simulink model "Voltage_and_Current_Measurement_MTL__18032026"  (R2024b)
settings: Solver=VariableStepAuto  StartTime=0.0  StopTime=10.0  RelTol=1e-3
libraries: spsThreePhaseVIMeasurementLib x12, spsRMSLib x8, spsThreePhasePISectionLineLib x6, spsThreePhaseSeriesRLCBranchLib x6, spsThreePhaseSourceLib x6, sps_lib x5, spsPower3phInstantaneousLib x4, spsGroundLib x3, spsThreePhaseSeriesRLCLoadLib x2, spsThreePhaseParallelRLCBranchLib x1
settings Model: Creator=cachu  LastModifiedBy=cachu

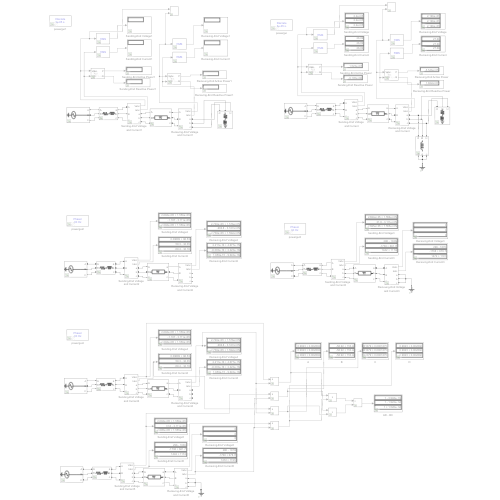
[thumbnail: Simulink's stored preview of the top-level diagram]
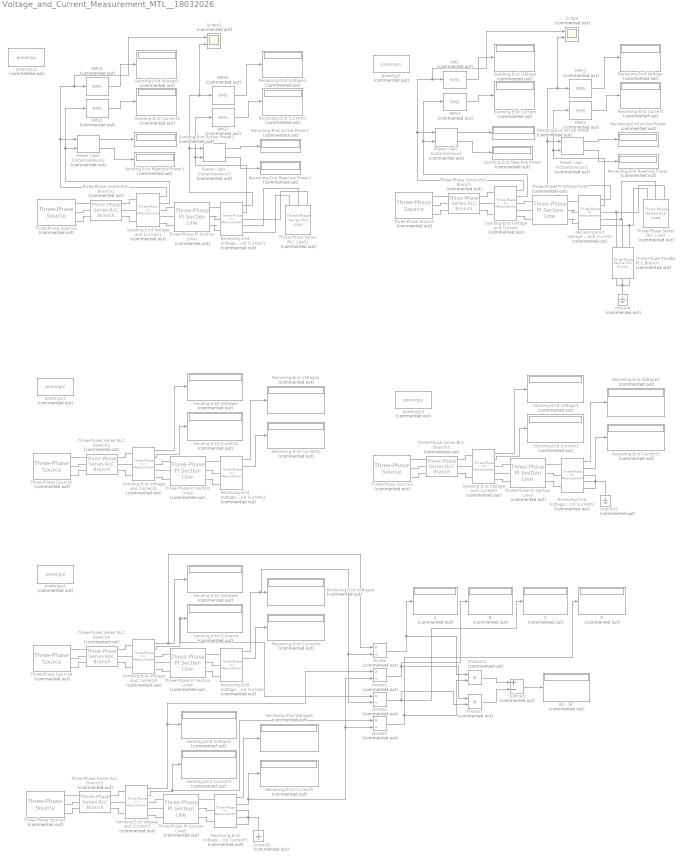
== system Voltage_and_Current_Measurement_MTL__18032026 ==
  A : Display  Commented=on
  AD - BC : Display  Commented=on
  B : Display  Commented=on
  C : Display  Commented=on
  D : Display  Commented=on
  Divide{,1..3} (4 alike) : Product  Commented=on  Inputs=*/
  Ground : spsGroundLib/Ground  Commented=on  LConnTagsString=a
  Ground1 : spsGroundLib/Ground  Commented=on  LConnTagsString=a
  Ground2 : spsGroundLib/Ground  Commented=on  LConnTagsString=a
  Power (3ph, Instantaneous){,1..3} (4 alike) : spsPower3phInstantaneousLib/Power (3ph, Instantaneous)  Commented=on
  Product : Product  Commented=on
  Product1 : Product  Commented=on
  RMS{,1..7} (8 alike) : spsRMSLib/RMS  Commented=on  TrueRMS=on  Freq=50  RMSInit=120  Ts=0
  Recieving-End Active Power : Display  Commented=on
  Recieving-End Active Power1 : Display  Commented=on
  Recieving-End Current{,1..5} (6 alike) : Display  Commented=on
  Recieving-End Reactive Power : Display  Commented=on
  Recieving-End Reactive Power1 : Display  Commented=on
  Recieving-End Voltage{,1..5} (6 alike) : Display  Commented=on
  Recieving-End Voltage and Current{,1,4..5} (4 alike) : spsThreePhaseVIMeasurementLib/Three-Phase V-I Measurement  Commented=on  VoltageMeasurement=phase-to-phase  SetLabelV=off  LabelV=Vabc  Vpu=off  VpuLL=off  CurrentMeasurement=yes  SetLabelI=off  LabelI=Iabc  Ipu=off  Pbase=100e6  Vbase=500e3  OutputType=Complex  PhasorSimulation=off  PSBequivalent=0
  Recieving-End Voltage and Current2 : spsThreePhaseVIMeasurementLib/Three-Phase V-I Measurement  Commented=on  VoltageMeasurement=phase-to-phase  SetLabelV=off  LabelV=Vabc  Vpu=off  VpuLL=off  CurrentMeasurement=yes  SetLabelI=off  LabelI=Iabc  Ipu=off  Pbase=100e6  Vbase=500e3  OutputType=Complex  PhasorSimulation=on  PSBequivalent=0
  Recieving-End Voltage and Current3 : spsThreePhaseVIMeasurementLib/Three-Phase V-I Measurement  Commented=on  VoltageMeasurement=phase-to-phase  SetLabelV=off  LabelV=Vabc  Vpu=off  VpuLL=off  CurrentMeasurement=yes  SetLabelI=off  LabelI=Iabc  Ipu=off  Pbase=100e6  Vbase=500e3  OutputType=Complex  PhasorSimulation=on  PSBequivalent=0
  Scope : Scope  Commented=on  NumInputPorts=2
  Scope1 : Scope  Commented=on  NumInputPorts=2
  Sending-End Active Power : Display  Commented=on
  Sending-End Active Power1 : Display  Commented=on
  Sending-End Current{,1..5} (6 alike) : Display  Commented=on
  Sending-End Reactive Power : Display  Commented=on
  Sending-End Reactive Power1 : Display  Commented=on
  Sending-End Voltage{,1..5} (6 alike) : Display  Commented=on
  Sending-End Voltage and Current{,1,4..5} (4 alike) : spsThreePhaseVIMeasurementLib/Three-Phase V-I Measurement  Commented=on  VoltageMeasurement=phase-to-phase  SetLabelV=off  LabelV=Vabc  Vpu=off  VpuLL=off  CurrentMeasurement=yes  SetLabelI=off  LabelI=Iabc  Ipu=off  Pbase=100e6  Vbase=500e3  OutputType=Complex  PhasorSimulation=off  PSBequivalent=0
  Sending-End Voltage and Current2 : spsThreePhaseVIMeasurementLib/Three-Phase V-I Measurement  Commented=on  VoltageMeasurement=phase-to-phase  SetLabelV=off  LabelV=Vabc  Vpu=off  VpuLL=off  CurrentMeasurement=yes  SetLabelI=off  LabelI=Iabc  Ipu=off  Pbase=100e6  Vbase=500e3  OutputType=Complex  PhasorSimulation=on  PSBequivalent=0
  Sending-End Voltage and Current3 : spsThreePhaseVIMeasurementLib/Three-Phase V-I Measurement  Commented=on  VoltageMeasurement=phase-to-phase  SetLabelV=off  LabelV=Vabc  Vpu=off  VpuLL=off  CurrentMeasurement=yes  SetLabelI=off  LabelI=Iabc  Ipu=off  Pbase=100e6  Vbase=500e3  OutputType=Complex  PhasorSimulation=on  PSBequivalent=0
  Subtract : Sum  Commented=on  Inputs=+-
  Three-Phase PI Section Line{,1..5} (6 alike) : spsThreePhasePISectionLineLib/Three-Phase PI Section Line  Commented=on  LConnTagsString=a|b|c  RConnTagsString=A|B|C  Length=150  Frequency=50  Resistances=[0.1 0.2]  Inductances=[2e-3 4e-3]  Capacitances=[8e-9 16e-9]
  Three-Phase Parallel RLC Branch : spsThreePhaseParallelRLCBranchLib/Three-Phase Parallel RLC Branch  Commented=on  LConnTagsString=A|B|C  RConnTagsString=A|B|C  BranchType=L  Resistance=0  Inductance=20  Capacitance=0  Measurements=None
  Three-Phase Series RLC Branch{,1..5} (6 alike) : spsThreePhaseSeriesRLCBranchLib/Three-Phase Series RLC Branch  Commented=on  LConnTagsString=A|B|C  RConnTagsString=A|B|C  BranchType=RL  Resistance=0.01  Inductance=1e-12  Capacitance=1e-6  Measurements=None
  Three-Phase Series RLC Load : spsThreePhaseSeriesRLCLoadLib/Three-Phase Series RLC Load  Commented=on  LConnTagsString=A|B|C  Configuration=Y (grounded)  NominalVoltage=220e3  Vabc=[1e3 1e3 1e3]  Vabcp=[1e3 1e3 1e3]  NominalFrequency=50  UnbalancedPower=off  ActivePower=5e6  InductivePower=1.6e6  CapacitivePower=0  Pabc=[10e3 9e3 11e3]  QLabc=[100 90 110]  QCabc=[100 90 110]  Pabcp=[10e3 9e3 11e3]  QLabcp=[100 90 110]  QCabcp=[100 90 110]  Measurements=None  LoadType=constant Z
  Three-Phase Series RLC Load1 : spsThreePhaseSeriesRLCLoadLib/Three-Phase Series RLC Load  Commented=on  LConnTagsString=A|B|C  Configuration=Y (grounded)  NominalVoltage=220e3  Vabc=[1e3 1e3 1e3]  Vabcp=[1e3 1e3 1e3]  NominalFrequency=50  UnbalancedPower=off  ActivePower=5e6  InductivePower=1.6e6  CapacitivePower=0  Pabc=[10e3 9e3 11e3]  QLabc=[100 90 110]  QCabc=[100 90 110]  Pabcp=[10e3 9e3 11e3]  QLabcp=[100 90 110]  QCabcp=[100 90 110]  Measurements=None  LoadType=constant Z
  Three-Phase Source{,1..5} (6 alike) : spsThreePhaseSourceLib/Three-Phase Source  Commented=on  InternalConnection=Yg  VoltagePhases=off  Voltage=220e3  PhaseAngle=0  Voltage_phases=[25e3 25e3 25e3]/sqrt(3)  PhaseAngles_phases=[0 -120 +120]  Frequency=50  NonIdealSource=off  SpecifyImpedance=off  Resistance=0.8929  Inductance=16.58e-3  ShortCircuitLevel=100e6  BaseVoltage=25e3  XRratio=7  BusType=swing  Pref=10e3  Qref=0  Prefabc=[10e3, 10e3, 10e3]  Qrefabc=[0, 0, 0]  Qmin=-inf  Qmax=inf
  powergui : sps_lib/powergui  Priority=1  Commented=on  SimulationMode=Discrete  SampleTime=50e-6  frequency=50  Iterations=50  frequencyindice=50  Pbase=100e6  ErrMax=1e-4  UnitsV=kV  UnitsW=MW  buscounter=0  FunctionMessages=off  echomessages=off  EnableUseOfTLC=off  CurrentSourceSwitches=off  DisableSnubberDevices=off  DisableRonSwitches=off  DisableVfSwitches=off  DisplayEquations=off  AutomaticDiscreteSolvers=off  SolverType=Tustin/Backward Euler (TBE)  Interpol=off  ExternalGateDelay=off  methode=off  Ts=100  x0status=blocks  SPID=on  SwTol=0  HookPort=off  NonlinearTolerance=1e-4  nMaxIteration=100  ContinueOnMaxIteration=off  RestoreLinks=warning  ResistiveCurrentMeasurement=off  Frange=[0:2:500]  Ylog=off  Xlog=on  ShowGrid=off  save=off  variable=ZData  structure=0  ZoomFFT=off  StartTime=0.0  cycles=1  DisplayStyle=1  fundamental=60  FreqAxis=off  MaxFrequency=1000  frequencyindicesteady=1  RmsSteady=1  display=off
  powergui1 : sps_lib/powergui  Priority=1  Commented=on  SimulationMode=Discrete  SampleTime=50e-6  frequency=50  Iterations=50  frequencyindice=50  Pbase=100e6  ErrMax=1e-4  UnitsV=kV  UnitsW=MW  buscounter=0  FunctionMessages=off  echomessages=off  EnableUseOfTLC=off  CurrentSourceSwitches=off  DisableSnubberDevices=off  DisableRonSwitches=off  DisableVfSwitches=off  DisplayEquations=off  AutomaticDiscreteSolvers=off  SolverType=Tustin/Backward Euler (TBE)  Interpol=off  ExternalGateDelay=off  methode=off  Ts=100  x0status=blocks  SPID=on  SwTol=0  HookPort=off  NonlinearTolerance=1e-4  nMaxIteration=100  ContinueOnMaxIteration=off  RestoreLinks=warning  ResistiveCurrentMeasurement=off  Frange=[0:2:500]  Ylog=off  Xlog=on  ShowGrid=off  save=off  variable=ZData  structure=0  ZoomFFT=off  StartTime=0.0  cycles=1  DisplayStyle=1  fundamental=60  FreqAxis=off  MaxFrequency=1000  frequencyindicesteady=1  RmsSteady=1  display=off
  powergui2 : sps_lib/powergui  Priority=1  Commented=on  SimulationMode=Phasor  SampleTime=50e-6  frequency=50  Iterations=50  frequencyindice=50  Pbase=100e6  ErrMax=1e-4  UnitsV=kV  UnitsW=MW  buscounter=0  FunctionMessages=off  echomessages=off  EnableUseOfTLC=off  CurrentSourceSwitches=off  DisableSnubberDevices=off  DisableRonSwitches=off  DisableVfSwitches=off  DisplayEquations=off  AutomaticDiscreteSolvers=off  SolverType=Tustin/Backward Euler (TBE)  Interpol=off  ExternalGateDelay=off  methode=off  Ts=100  x0status=blocks  SPID=on  SwTol=0  HookPort=off  NonlinearTolerance=1e-4  nMaxIteration=100  ContinueOnMaxIteration=off  RestoreLinks=warning  ResistiveCurrentMeasurement=off  Frange=[0:2:500]  Ylog=off  Xlog=on  ShowGrid=off  save=off  variable=ZData  structure=0  ZoomFFT=off  StartTime=0.0  cycles=1  DisplayStyle=1  fundamental=60  FreqAxis=off  MaxFrequency=1000  frequencyindicesteady=1  RmsSteady=1  display=off
  powergui3 : sps_lib/powergui  Priority=1  Commented=on  SimulationMode=Phasor  SampleTime=50e-6  frequency=50  Iterations=50  frequencyindice=50  Pbase=100e6  ErrMax=1e-4  UnitsV=kV  UnitsW=MW  buscounter=0  FunctionMessages=off  echomessages=off  EnableUseOfTLC=off  CurrentSourceSwitches=off  DisableSnubberDevices=off  DisableRonSwitches=off  DisableVfSwitches=off  DisplayEquations=off  AutomaticDiscreteSolvers=off  SolverType=Tustin/Backward Euler (TBE)  Interpol=off  ExternalGateDelay=off  methode=off  Ts=100  x0status=blocks  SPID=on  SwTol=0  HookPort=off  NonlinearTolerance=1e-4  nMaxIteration=100  ContinueOnMaxIteration=off  RestoreLinks=warning  ResistiveCurrentMeasurement=off  Frange=[0:2:500]  Ylog=off  Xlog=on  ShowGrid=off  save=off  variable=ZData  structure=0  ZoomFFT=off  StartTime=0.0  cycles=1  DisplayStyle=1  fundamental=60  FreqAxis=off  MaxFrequency=1000  frequencyindicesteady=1  RmsSteady=1  display=off
  powergui4 : sps_lib/powergui  Priority=1  Commented=on  SimulationMode=Phasor  SampleTime=50e-6  frequency=50  Iterations=50  frequencyindice=50  Pbase=100e6  ErrMax=1e-4  UnitsV=kV  UnitsW=MW  buscounter=0  FunctionMessages=off  echomessages=off  EnableUseOfTLC=off  CurrentSourceSwitches=off  DisableSnubberDevices=off  DisableRonSwitches=off  DisableVfSwitches=off  DisplayEquations=off  AutomaticDiscreteSolvers=off  SolverType=Tustin/Backward Euler (TBE)  Interpol=off  ExternalGateDelay=off  methode=off  Ts=100  x0status=blocks  SPID=on  SwTol=0  HookPort=off  NonlinearTolerance=1e-4  nMaxIteration=100  ContinueOnMaxIteration=off  RestoreLinks=warning  ResistiveCurrentMeasurement=off  Frange=[0:2:500]  Ylog=off  Xlog=on  ShowGrid=off  save=off  variable=ZData  structure=0  ZoomFFT=off  StartTime=0.0  cycles=1  DisplayStyle=1  fundamental=60  FreqAxis=off  MaxFrequency=1000  frequencyindicesteady=1  RmsSteady=1  display=off
  wires:
  RMS/1 -> Sending-End Voltage/1
  Sending-End Voltage and Current/1 -> "Power (3ph, Instantaneous)"/1, Scope/1, RMS/1
  Sending-End Voltage and Current/2 -> RMS1/1, "Power (3ph, Instantaneous)"/2
  RMS1/1 -> Sending-End Current/1
  "Power (3ph, Instantaneous)"/2 -> Sending-End Reactive Power/1
  "Power (3ph, Instantaneous)"/1 -> Sending-End Active Power/1
  Recieving-End Voltage and Current/1 -> Scope/2, RMS2/1, "Power (3ph, Instantaneous)1"/1
  Recieving-End Voltage and Current/2 -> RMS3/1, "Power (3ph, Instantaneous)1"/2
  "Power (3ph, Instantaneous)1"/1 -> Recieving-End Active Power/1
  RMS3/1 -> Recieving-End Current/1
  RMS2/1 -> Recieving-End Voltage/1
  "Power (3ph, Instantaneous)1"/2 -> Recieving-End Reactive Power/1
  Sending-End Voltage and Current1/1 -> "Power (3ph, Instantaneous)2"/1, Scope1/1, RMS4/1
  Recieving-End Voltage and Current1/1 -> Scope1/2, RMS6/1, "Power (3ph, Instantaneous)3"/1
  "Power (3ph, Instantaneous)2"/1 -> Sending-End Active Power1/1
  RMS4/1 -> Sending-End Voltage1/1
  "Power (3ph, Instantaneous)2"/2 -> Sending-End Reactive Power1/1
  RMS7/1 -> Recieving-End Current1/1
  RMS6/1 -> Recieving-End Voltage1/1
  Recieving-End Voltage and Current1/2 -> RMS7/1, "Power (3ph, Instantaneous)3"/2
  "Power (3ph, Instantaneous)3"/2 -> Recieving-End Reactive Power1/1
  "Power (3ph, Instantaneous)3"/1 -> Recieving-End Active Power1/1
  Sending-End Voltage and Current1/2 -> RMS5/1, "Power (3ph, Instantaneous)2"/2
  RMS5/1 -> Sending-End Current1/1
  Recieving-End Voltage and Current2/1 -> Recieving-End Voltage2/1
  Recieving-End Voltage and Current2/2 -> Recieving-End Current2/1
  Sending-End Voltage and Current2/1 -> Sending-End Voltage2/1
  Sending-End Voltage and Current2/2 -> Sending-End Current2/1
  Recieving-End Voltage and Current3/1 -> Recieving-End Voltage3/1
  Recieving-End Voltage and Current3/2 -> Recieving-End Current3/1
  Sending-End Voltage and Current3/2 -> Sending-End Current3/1
  Sending-End Voltage and Current3/1 -> Sending-End Voltage3/1
  Sending-End Voltage and Current5/1 -> Divide1/1, Sending-End Voltage5/1
  Sending-End Voltage and Current5/2 -> Divide3/1, Sending-End Current5/1
  Recieving-End Voltage and Current4/1 -> Divide2/2, Divide/2, Recieving-End Voltage4/1
  Recieving-End Voltage and Current4/2 -> Recieving-End Current4/1
  Sending-End Voltage and Current4/2 -> Divide2/1, Sending-End Current4/1
  Sending-End Voltage and Current4/1 -> Divide/1, Sending-End Voltage4/1
  Recieving-End Voltage and Current5/1 -> Recieving-End Voltage5/1
  Recieving-End Voltage and Current5/2 -> Divide1/2, Divide3/2, Recieving-End Current5/1
  Divide/1 -> Product1/1, A/1
  Divide1/1 -> Product/1, B/1
  Divide2/1 -> Product/2, C/1
  Divide3/1 -> Product1/2, D/1
  Subtract/1 -> AD - BC/1
  Product1/1 -> Subtract/1
  Product/1 -> Subtract/2
  connections:
  Sending-End Voltage and Current/RConn1 -- Three-Phase PI Section Line/LConn1
  Sending-End Voltage and Current/RConn2 -- Three-Phase PI Section Line/LConn2
  Sending-End Voltage and Current/RConn3 -- Three-Phase PI Section Line/LConn3
  Recieving-End Voltage and Current/LConn1 -- Three-Phase PI Section Line/RConn1
  Three-Phase PI Section Line/RConn2 -- Recieving-End Voltage and Current/LConn2
  Three-Phase PI Section Line/RConn3 -- Recieving-End Voltage and Current/LConn3
  Three-Phase Series RLC Load/LConn1 -- Recieving-End Voltage and Current/RConn3 -- Three-Phase Parallel RLC Branch/LConn3
  Recieving-End Voltage and Current/RConn2 -- Three-Phase Parallel RLC Branch/LConn2 -- Three-Phase Series RLC Load/LConn2
  Three-Phase Series RLC Load/LConn3 -- Recieving-End Voltage and Current/RConn1 -- Three-Phase Parallel RLC Branch/LConn1
  Three-Phase Source/RConn1 -- Three-Phase Series RLC Branch/LConn1
  Three-Phase Series RLC Branch/LConn2 -- Three-Phase Source/RConn2
  Three-Phase Series RLC Branch/LConn3 -- Three-Phase Source/RConn3
  Three-Phase Series RLC Branch/RConn1 -- Sending-End Voltage and Current/LConn1
  Sending-End Voltage and Current/LConn2 -- Three-Phase Series RLC Branch/RConn2
  Three-Phase Series RLC Branch/RConn3 -- Sending-End Voltage and Current/LConn3
  Ground/LConn1 -- Three-Phase Parallel RLC Branch/RConn1 -- Three-Phase Parallel RLC Branch/RConn3 -- Three-Phase Parallel RLC Branch/RConn2
  Three-Phase Series RLC Load1/LConn1 -- Recieving-End Voltage and Current1/RConn3
  Recieving-End Voltage and Current1/RConn2 -- Three-Phase Series RLC Load1/LConn2
  Three-Phase Series RLC Load1/LConn3 -- Recieving-End Voltage and Current1/RConn1
  Three-Phase Series RLC Branch1/RConn1 -- Sending-End Voltage and Current1/LConn1
  Three-Phase Source1/RConn1 -- Three-Phase Series RLC Branch1/LConn1
  Three-Phase Series RLC Branch1/LConn2 -- Three-Phase Source1/RConn2
  Sending-End Voltage and Current1/RConn2 -- Three-Phase PI Section Line1/LConn2
  Sending-End Voltage and Current1/RConn1 -- Three-Phase PI Section Line1/LConn1
  Three-Phase PI Section Line1/RConn2 -- Recieving-End Voltage and Current1/LConn2
  Three-Phase PI Section Line1/RConn3 -- Recieving-End Voltage and Current1/LConn3
  Sending-End Voltage and Current1/RConn3 -- Three-Phase PI Section Line1/LConn3
  Three-Phase Series RLC Branch1/RConn3 -- Sending-End Voltage and Current1/LConn3
  Sending-End Voltage and Current1/LConn2 -- Three-Phase Series RLC Branch1/RConn2
  Recieving-End Voltage and Current1/LConn1 -- Three-Phase PI Section Line1/RConn1
  Three-Phase Series RLC Branch1/LConn3 -- Three-Phase Source1/RConn3
  Sending-End Voltage and Current2/LConn2 -- Three-Phase Series RLC Branch2/RConn2
  Three-Phase Source2/RConn1 -- Three-Phase Series RLC Branch2/LConn1
  Three-Phase Series RLC Branch2/LConn2 -- Three-Phase Source2/RConn2
  Three-Phase Series RLC Branch2/RConn3 -- Sending-End Voltage and Current2/LConn3
  Sending-End Voltage and Current2/RConn2 -- Three-Phase PI Section Line2/LConn2
  Sending-End Voltage and Current2/RConn1 -- Three-Phase PI Section Line2/LConn1
  Sending-End Voltage and Current2/RConn3 -- Three-Phase PI Section Line2/LConn3
  Three-Phase Series RLC Branch2/RConn1 -- Sending-End Voltage and Current2/LConn1
  Three-Phase PI Section Line2/RConn2 -- Recieving-End Voltage and Current2/LConn2
  Three-Phase PI Section Line2/RConn3 -- Recieving-End Voltage and Current2/LConn3
  Three-Phase Series RLC Branch2/LConn3 -- Three-Phase Source2/RConn3
  Recieving-End Voltage and Current2/LConn1 -- Three-Phase PI Section Line2/RConn1
  Three-Phase PI Section Line3/RConn3 -- Recieving-End Voltage and Current3/LConn3
  Sending-End Voltage and Current3/RConn2 -- Three-Phase PI Section Line3/LConn2
  Sending-End Voltage and Current3/RConn1 -- Three-Phase PI Section Line3/LConn1
  Three-Phase Series RLC Branch3/LConn2 -- Three-Phase Source3/RConn2
  Three-Phase Series RLC Branch3/RConn1 -- Sending-End Voltage and Current3/LConn1
  Three-Phase Source3/RConn1 -- Three-Phase Series RLC Branch3/LConn1
  Three-Phase PI Section Line3/RConn2 -- Recieving-End Voltage and Current3/LConn2
  Sending-End Voltage and Current3/RConn3 -- Three-Phase PI Section Line3/LConn3
  Sending-End Voltage and Current3/LConn2 -- Three-Phase Series RLC Branch3/RConn2
  Three-Phase Series RLC Branch3/LConn3 -- Three-Phase Source3/RConn3
  Three-Phase Series RLC Branch3/RConn3 -- Sending-End Voltage and Current3/LConn3
  Recieving-End Voltage and Current3/LConn1 -- Three-Phase PI Section Line3/RConn1
  Recieving-End Voltage and Current3/RConn1 -- Ground1/LConn1 -- Recieving-End Voltage and Current3/RConn3 -- Recieving-End Voltage and Current3/RConn2
  Recieving-End Voltage and Current5/RConn2 -- Ground2/LConn1 -- Recieving-End Voltage and Current5/RConn1 -- Recieving-End Voltage and Current5/RConn3
  Sending-End Voltage and Current4/RConn2 -- Three-Phase PI Section Line4/LConn2
  Recieving-End Voltage and Current5/LConn1 -- Three-Phase PI Section Line5/RConn1
  Sending-End Voltage and Current5/RConn3 -- Three-Phase PI Section Line5/LConn3
  Three-Phase Series RLC Branch5/LConn3 -- Three-Phase Source5/RConn3
  Three-Phase Series RLC Branch4/LConn2 -- Three-Phase Source4/RConn2
  Three-Phase PI Section Line5/RConn2 -- Recieving-End Voltage and Current5/LConn2
  Sending-End Voltage and Current5/RConn2 -- Three-Phase PI Section Line5/LConn2
  Three-Phase PI Section Line5/RConn3 -- Recieving-End Voltage and Current5/LConn3
  Three-Phase Series RLC Branch5/LConn2 -- Three-Phase Source5/RConn2
  Three-Phase Series RLC Branch5/RConn1 -- Sending-End Voltage and Current5/LConn1
  Sending-End Voltage and Current5/RConn1 -- Three-Phase PI Section Line5/LConn1
  Three-Phase Series RLC Branch5/RConn3 -- Sending-End Voltage and Current5/LConn3
  Three-Phase Series RLC Branch4/RConn1 -- Sending-End Voltage and Current4/LConn1
  Sending-End Voltage and Current4/RConn3 -- Three-Phase PI Section Line4/LConn3
  Recieving-End Voltage and Current4/LConn1 -- Three-Phase PI Section Line4/RConn1
  Three-Phase Source5/RConn1 -- Three-Phase Series RLC Branch5/LConn1
  Sending-End Voltage and Current4/RConn1 -- Three-Phase PI Section Line4/LConn1
  Three-Phase Series RLC Branch4/LConn3 -- Three-Phase Source4/RConn3
  Sending-End Voltage and Current4/LConn2 -- Three-Phase Series RLC Branch4/RConn2
  Three-Phase PI Section Line4/RConn3 -- Recieving-End Voltage and Current4/LConn3
  Three-Phase PI Section Line4/RConn2 -- Recieving-End Voltage and Current4/LConn2
  Three-Phase Series RLC Branch4/RConn3 -- Sending-End Voltage and Current4/LConn3
  Sending-End Voltage and Current5/LConn2 -- Three-Phase Series RLC Branch5/RConn2
  Three-Phase Source4/RConn1 -- Three-Phase Series RLC Branch4/LConn1
